simulink model "Position"  (R2021a)
settings: Solver=ode113  StartTime=0.0  StopTime=1  RelTol=1e-6
model workspace (MAT data in the model file):
  Vdc = 30
  f_pwm = 10000
libraries: pid_lib x3, spsControlledVoltageSourceLib x1, spsGroundLib x1, cstblocks x1, spsPermanentMagnetSynchronousMachineLib x1, spsThreePhaseVIMeasurementLib x1, spsUniversalBridgeLib x1, spsTriangleGeneratorLib x1, spspowerguiLib x1
settings Model: SimulationMode=accelerator  Creator=Zzx  LastModifiedBy=Zzx
settings SolverCC: ZeroCrossAlgorithm=Adaptive

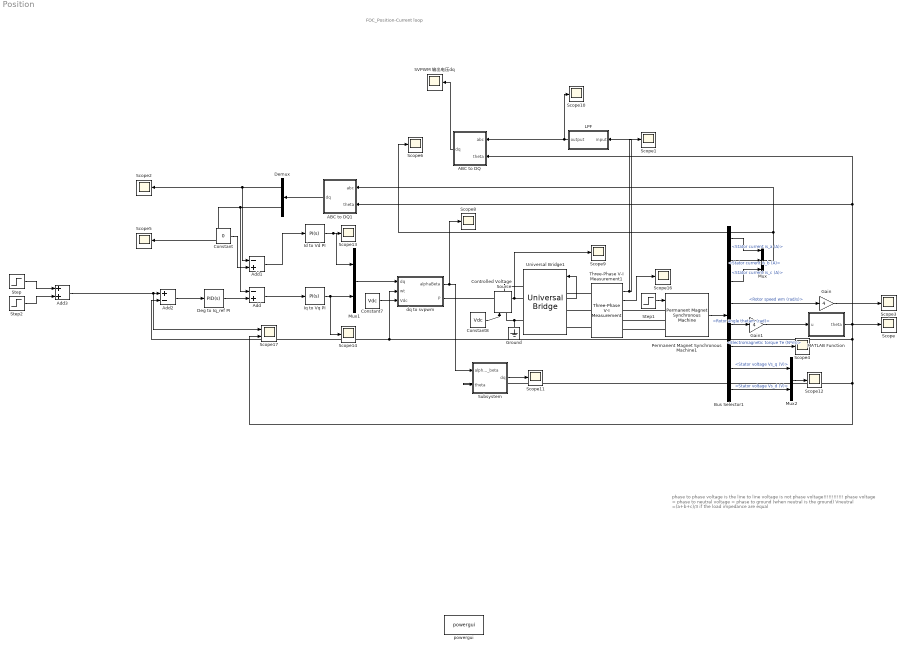
== system Position ==
  note: FOC_Position-Current loop
  note: phase to phase voltage is the line to line voltage
      | is not phase voltage!!!!!!!!!!!!
      | phase voltage = phase to neutral voltage = phase to ground (when neutral is the ground)
      | Vneutral =(a+b+c)/3 if the load impedance are equal
  ABC to DQ : Subsystem
  ABC to DQ1 : Subsystem
  Add : Sum  Inputs=-+
  Add1 : Sum  Inputs=-+
  Add2 : Sum  Inputs=+-
  Add3 : Sum
  Bus Selector1 : BusSelector  OutputSignals=Stator current is_a (A),Stator current is_b (A),Stator current is_c (A),Rotor speed wm (rad/s),Rotor angle thetam (rad),Electromagnetic torque Te (N*m),Stator voltage Vs_q (V),Stator voltage Vs_d (V)
  Constant : Constant  Value=0
  Constant7 : Constant  Value=Vdc
  Constant8 : Constant  Value=Vdc
  Controlled Voltage Source : spsControlledVoltageSourceLib/Controlled Voltage Source  Initialize=on  Source_Type=DC  Amplitude=0  Phase=0  Frequency=0  Measurements=Voltage
  Deg to Iq_ref PI : pid_lib/PID Controller  Controller=PID  Form=Parallel  TimeDomain=Continuous-time  UseExternalTs=off  SampleTime=-1  IntegratorMethod=Forward Euler  FilterMethod=Forward Euler  ControllerParametersSource=internal  P=20  I=0  D=1  UseFilter=on  N=70  TunerSelectOption=Frequency Response Based  InitialConditionSource=internal  InitialConditionForIntegrator=0  InitialConditionForFilter=0  DifferentiatorICPrevScaledInput=0  ExternalReset=none  TrackingMode=off  Kt=1  LimitOutput=off  SatLimitsSource=internal  UpperSaturationLimit=inf  LowerSaturationLimit=-inf  LinearizeAsGain=on  AntiWindupMode=none  Kb=1  POutMin=[]  POutMax=[]  IOutMin=[]  IOutMax=[]  DOutMin=[]  DOutMax=[]  NOutMin=[]  NOutMax=[]  SumOutMin=[]  SumOutMax=[]  SaturationOutMin=[]  SaturationOutMax=[]  PParamMin=[]  PParamMax=[]  IParamMin=[]  IParamMax=[]  DParamMin=[]  DParamMax=[]  NParamMin=[]  NParamMax=[]  KbParamMin=[]  KbParamMax=[]  KtParamMin=[]  KtParamMax=[]  KbOutMin=[]  KbOutMax=[]  KtOutMin=[]  KtOutMax=[]  IntegratorOutMin=[]  IntegratorOutMax=[]  FilterOutMin=[]  FilterOutMax=[]  SumI1OutMin=[]  SumI1OutMax=[]  SumI2OutMin=[]  SumI2OutMax=[]  SumI3OutMin=[]  SumI3OutMax=[]  SumI4OutMin=[]  SumI4OutMax=[]  SumDOutMin=[]  SumDOutMax=[]  DifferentiatorOutMin=[]  DifferentiatorOutMax=[]  FilterDiffOutCoefMin=[]  FilterDiffOutCoefMax=[]  ReciprocalOutMin=[]  ReciprocalOutMax=[]  SumDenOutMin=[]  SumDenOutMax=[]  SumNumOutMin=[]  SumNumOutMax=[]  DivideOutMin=[]  DivideOutMax=[]  UdiffTsProdOutMin=[]  UdiffTsProdOutMax=[]  NTsProdOutMin=[]  NTsProdOutMax=[]  UintegralTsProdOutMin=[]  UintegralTsProdOutMax=[]  UngainTsProdOutMin=[]  UngainTsProdOutMax=[]  IntegratorContinuousStateAttributes=''  IntegratorStateMustResolveToSignalObject=off  IntegratorRTWStateStorageClass=Auto  FilterContinuousStateAttributes=''  FilterStateMustResolveToSignalObject=off  FilterRTWStateStorageClass=Auto  ParallelPVariant=InternalParameters  IdealPVariant=Disabled  IVariant=InternalParameters  DVariant=InternalParameters  IntegratorVariant=Continuous  SatVariant=Disabled  AWVariant=Passthrough  PCopyVariant=Disabled  TRVariant=Disabled  FdbkBlocksVariant=Forward  IdealPFdbkVariant=Disabled  SatFdbkVariant=Disabled  DerivativeFilterVariant=ContFilter  NVariant=InternalParameters  NCopyVariant=Disabled  FilterICVariant=InternalICsFilter  IntegratorICVariant=InternalICs  ExternalResetVariant=Disabled  TRSumVariant=Passthrough  SumFdbkVariant=Disabled  SumVariant=Sum_PID  TsampFilterVariant=InternalTs  TsampNgainVariant=Passthrough  TsampIntegralVariant=Passthrough  ExternalSaturationOutDataTypeStr=Inherit: Same as second input
  Demux : Demux  Outputs=2
  Gain : Gain  Gain=4
  Gain1 : Gain  Gain=4
  Ground : spsGroundLib/Ground  LConnTagsString=a
  Id to Vd PI : pid_lib/PID Controller  Controller=PI  Form=Parallel  TimeDomain=Continuous-time  UseExternalTs=off  SampleTime=-1  IntegratorMethod=Forward Euler  FilterMethod=Forward Euler  ControllerParametersSource=internal  P=10  I=0.1  D=0  UseFilter=on  N=100  TunerSelectOption=Transfer Function Based (PID Tuner App)  InitialConditionSource=internal  InitialConditionForIntegrator=0  InitialConditionForFilter=0  DifferentiatorICPrevScaledInput=0  ExternalReset=none  TrackingMode=off  Kt=1  LimitOutput=off  SatLimitsSource=internal  UpperSaturationLimit=inf  LowerSaturationLimit=-inf  LinearizeAsGain=on  AntiWindupMode=none  Kb=1  POutMin=[]  POutMax=[]  IOutMin=[]  IOutMax=[]  DOutMin=[]  DOutMax=[]  NOutMin=[]  NOutMax=[]  SumOutMin=[]  SumOutMax=[]  SaturationOutMin=[]  SaturationOutMax=[]  PParamMin=[]  PParamMax=[]  IParamMin=[]  IParamMax=[]  DParamMin=[]  DParamMax=[]  NParamMin=[]  NParamMax=[]  KbParamMin=[]  KbParamMax=[]  KtParamMin=[]  KtParamMax=[]  KbOutMin=[]  KbOutMax=[]  KtOutMin=[]  KtOutMax=[]  IntegratorOutMin=[]  IntegratorOutMax=[]  FilterOutMin=[]  FilterOutMax=[]  SumI1OutMin=[]  SumI1OutMax=[]  SumI2OutMin=[]  SumI2OutMax=[]  SumI3OutMin=[]  SumI3OutMax=[]  SumI4OutMin=[]  SumI4OutMax=[]  SumDOutMin=[]  SumDOutMax=[]  DifferentiatorOutMin=[]  DifferentiatorOutMax=[]  FilterDiffOutCoefMin=[]  FilterDiffOutCoefMax=[]  ReciprocalOutMin=[]  ReciprocalOutMax=[]  SumDenOutMin=[]  SumDenOutMax=[]  SumNumOutMin=[]  SumNumOutMax=[]  DivideOutMin=[]  DivideOutMax=[]  UdiffTsProdOutMin=[]  UdiffTsProdOutMax=[]  NTsProdOutMin=[]  NTsProdOutMax=[]  UintegralTsProdOutMin=[]  UintegralTsProdOutMax=[]  UngainTsProdOutMin=[]  UngainTsProdOutMax=[]  IntegratorContinuousStateAttributes=''  IntegratorStateMustResolveToSignalObject=off  IntegratorRTWStateStorageClass=Auto  FilterContinuousStateAttributes=''  FilterStateMustResolveToSignalObject=off  FilterRTWStateStorageClass=Auto  ParallelPVariant=InternalParameters  IdealPVariant=Disabled  IVariant=InternalParameters  DVariant=Disabled  IntegratorVariant=Continuous  SatVariant=Disabled  AWVariant=Passthrough  PCopyVariant=Disabled  TRVariant=Disabled  FdbkBlocksVariant=Forward  IdealPFdbkVariant=Disabled  SatFdbkVariant=Disabled  DerivativeFilterVariant=Disabled  NVariant=Disabled  NCopyVariant=Disabled_SignalSpec  FilterICVariant=Disabled  IntegratorICVariant=InternalICs  ExternalResetVariant=Disabled  TRSumVariant=Passthrough  SumFdbkVariant=Disabled  SumVariant=Sum_PI  TsampFilterVariant=InternalTs  TsampNgainVariant=Passthrough  TsampIntegralVariant=Passthrough  ExternalSaturationOutDataTypeStr=Inherit: Same as second input
  Iq to Vq PI : pid_lib/PID Controller  Controller=PI  Form=Parallel  TimeDomain=Continuous-time  UseExternalTs=off  SampleTime=-1  IntegratorMethod=Forward Euler  FilterMethod=Forward Euler  ControllerParametersSource=internal  P=10  I=0.1  D=0  UseFilter=on  N=100  TunerSelectOption=Frequency Response Based  InitialConditionSource=internal  InitialConditionForIntegrator=0  InitialConditionForFilter=0  DifferentiatorICPrevScaledInput=0  ExternalReset=none  TrackingMode=off  Kt=1  LimitOutput=off  SatLimitsSource=internal  UpperSaturationLimit=inf  LowerSaturationLimit=-inf  LinearizeAsGain=on  AntiWindupMode=none  Kb=1  POutMin=[]  POutMax=[]  IOutMin=[]  IOutMax=[]  DOutMin=[]  DOutMax=[]  NOutMin=[]  NOutMax=[]  SumOutMin=[]  SumOutMax=[]  SaturationOutMin=[]  SaturationOutMax=[]  PParamMin=[]  PParamMax=[]  IParamMin=[]  IParamMax=[]  DParamMin=[]  DParamMax=[]  NParamMin=[]  NParamMax=[]  KbParamMin=[]  KbParamMax=[]  KtParamMin=[]  KtParamMax=[]  KbOutMin=[]  KbOutMax=[]  KtOutMin=[]  KtOutMax=[]  IntegratorOutMin=[]  IntegratorOutMax=[]  FilterOutMin=[]  FilterOutMax=[]  SumI1OutMin=[]  SumI1OutMax=[]  SumI2OutMin=[]  SumI2OutMax=[]  SumI3OutMin=[]  SumI3OutMax=[]  SumI4OutMin=[]  SumI4OutMax=[]  SumDOutMin=[]  SumDOutMax=[]  DifferentiatorOutMin=[]  DifferentiatorOutMax=[]  FilterDiffOutCoefMin=[]  FilterDiffOutCoefMax=[]  ReciprocalOutMin=[]  ReciprocalOutMax=[]  SumDenOutMin=[]  SumDenOutMax=[]  SumNumOutMin=[]  SumNumOutMax=[]  DivideOutMin=[]  DivideOutMax=[]  UdiffTsProdOutMin=[]  UdiffTsProdOutMax=[]  NTsProdOutMin=[]  NTsProdOutMax=[]  UintegralTsProdOutMin=[]  UintegralTsProdOutMax=[]  UngainTsProdOutMin=[]  UngainTsProdOutMax=[]  IntegratorContinuousStateAttributes=''  IntegratorStateMustResolveToSignalObject=off  IntegratorRTWStateStorageClass=Auto  FilterContinuousStateAttributes=''  FilterStateMustResolveToSignalObject=off  FilterRTWStateStorageClass=Auto  ParallelPVariant=InternalParameters  IdealPVariant=Disabled  IVariant=InternalParameters  DVariant=Disabled  IntegratorVariant=Continuous  SatVariant=Disabled  AWVariant=Passthrough  PCopyVariant=Disabled  TRVariant=Disabled  FdbkBlocksVariant=Forward  IdealPFdbkVariant=Disabled  SatFdbkVariant=Disabled  DerivativeFilterVariant=Disabled  NVariant=Disabled  NCopyVariant=Disabled_SignalSpec  FilterICVariant=Disabled  IntegratorICVariant=InternalICs  ExternalResetVariant=Disabled  TRSumVariant=Passthrough  SumFdbkVariant=Disabled  SumVariant=Sum_PI  TsampFilterVariant=InternalTs  TsampNgainVariant=Passthrough  TsampIntegralVariant=Passthrough  ExternalSaturationOutDataTypeStr=Inherit: Same as second input
  LPF : Subsystem
  MATLAB Function : MATLAB Function  TreatAsAtomicUnit=on
  Mux : Mux  Inputs=3
  Mux1 : Mux  Inputs=2
  Mux2 : Mux  Inputs=2
  Permanent Magnet Synchronous Machine1 : spsPermanentMagnetSynchronousMachineLib/Permanent Magnet Synchronous Machine  NbPhases=3  FluxDistribution=Sinusoidal  RotorType=Round  MechanicalLoad=Torque Tm  PresetModel=No  ShowDetailedParameters=on  MeasurementBus=off  Resistance=0.89  Inductance=8.5e-3  dqInductances=[8.5e-3,8.5e-3]  La=0.00062  MachineConstant=Voltage Constant (V_peak L-L / krpm)  Flux=0.0056925  VoltageCst=4.13  TorqueCst=0.034155  Flat=120  Mechanical=[ 0.8e-3, 0 4]  PolePairs=4  InitialConditions=[0,0, 0,0]  InitialConditions5ph=[0 0 0 0 0 0]  RefAngle=Aligned with phase A axis (original Park)  IterativeDiscreteModel=Trapezoidal non iterative  TsBlock=-1  TsPowergui=0
  SVPWM 输出电压dq : Scope
  Scope{,1..6,8..14,16} (15 alike) : Scope
  Scope17 : Scope  NumInputPorts=2
  Step : Step  Time=0.25  Before=1  After=5  SampleTime=0
  Step1 : Step  Time=0.5  After=0  SampleTime=0
  Step2 : Step  Time=0.75  After=-2  SampleTime=0
  Subsystem : Subsystem
  Three-Phase V-I Measurement1 : spsThreePhaseVIMeasurementLib/Three-Phase V-I Measurement  VoltageMeasurement=phase-to-ground  SetLabelV=off  LabelV=Vabc  Vpu=off  VpuLL=off  CurrentMeasurement=yes  SetLabelI=off  LabelI=Iabc  Ipu=off  Pbase=100e6  Vbase=500e3  OutputType=Complex  PhasorSimulation=off  PSBequivalent=0
  Universal Bridge1 : spsUniversalBridgeLib/Universal Bridge  Arms=3  SnubberResistance=1e5  SnubberCapacitance=inf  Device=IGBT / Diodes  Ron=1e-3  Lon=0  ForwardVoltages="[  0  0  ]"  ForwardVoltage=0  GTOparameters=[ 10e-6 , 20e-6 ]  IGBTparameters=[ 1e-6 , 2e-6 ]  Measurements=None  Measurements_2=None  converterType=Rectifier
  dq to svpwm : Subsystem
  powergui : spspowerguiLib/powergui  Priority=1  SimulationMode=Continuous  SampleTime=50e-6  frequency=60  Iterations=50  frequencyindice=0  Pbase=100e6  ErrMax=1e-4  UnitsV=kV  UnitsW=MW  buscounter=0  FunctionMessages=off  echomessages=off  EnableUseOfTLC=off  CurrentSourceSwitches=off  DisableSnubberDevices=off  DisableRonSwitches=off  DisableVfSwitches=off  DisplayEquations=off  AutomaticDiscreteSolvers=off  SolverType=Tustin/Backward Euler (TBE)  Interpol=off  ExternalGateDelay=off  methode=off  Ts=100  x0status=blocks  SPID=on  SwTol=0  HookPort=off  NonlinearTolerance=1e-4  nMaxIteration=100  ContinueOnMaxIteration=off  RestoreLinks=warning  ResistiveCurrentMeasurement=off  Frange=[0:2:500]  Ylog=off  Xlog=on  ShowGrid=off  save=off  variable=ZData  structure=0  ZoomFFT=off  StartTime=0.0  cycles=1  DisplayStyle=1  fundamental=60  FreqAxis=off  MaxFrequency=1000  frequencyindicesteady=1  RmsSteady=1  display=off
  wires:
  Three-Phase V-I Measurement1/1 -> LPF/1(input), Scope1/1
  Permanent Magnet Synchronous Machine1/1 -> Bus Selector1/1
  Bus Selector1/1 -> Mux/1  "<Stator current is_a (A)>"
  Bus Selector1/2 -> Mux/2  "<Stator current is_b (A)>"
  Bus Selector1/3 -> Mux/3  "<Stator current is_c (A)>"
  Mux/1 -> Scope6/1, ABC to DQ1/1(abc)
  Bus Selector1/5 -> Gain1/1  "<Rotor angle thetam (rad)>"
  ABC to DQ1/1(dq) -> Demux/1
  Constant/1 -> Add1/2
  Demux/1 -> Scope2/1, Add1/1
  Demux/2 -> Scope5/1, Add/1
  Bus Selector1/4 -> Gain/1  "<Rotor speed wm (rad/s)>"
  Bus Selector1/6 -> Scope4/1  "<Electromagnetic torque Te (N*m)>"
  Add1/1 -> Id to Vd PI/1
  dq to svpwm/2(P) -> Universal Bridge1/1, Scope9/1
  Mux1/1 -> dq to svpwm/1(dq)
  dq to svpwm/1(alphaBeta) -> Subsystem/1(alpha_beta), Scope8/1
  Bus Selector1/7 -> Mux2/1  "<Stator voltage Vs_q (V)>"
  Bus Selector1/8 -> Mux2/2  "<Stator voltage Vs_d (V)>"
  Mux2/1 -> Scope12/1
  Step1/1 -> Permanent Magnet Synchronous Machine1/1
  Constant7/1 -> dq to svpwm/3(Vdc)
  Three-Phase V-I Measurement1/2 -> Scope16/1
  Constant8/1 -> Controlled Voltage Source/1
  ABC to DQ/1(dq) -> SVPWM 输出电压dq/1
  Id to Vd PI/1 -> Mux1/1, Scope13/1
  Subsystem/1(dq) -> Scope11/1
  LPF/1(output) -> Scope10/1, ABC to DQ/1(abc)
  MATLAB Function/1(theta) -> Scope17/2, Subsystem/2(theta), Add2/2, dq to svpwm/2(wt), ABC to DQ1/2(theta), ABC to DQ/2(theta), Scope/1
  Add3/1 -> Scope17/1, Add2/1
  Step2/1 -> Add3/2
  Step/1 -> Add3/1
  Iq to Vq PI/1 -> Scope14/1, Mux1/2
  Add/1 -> Iq to Vq PI/1
  Gain/1 -> Scope3/1
  Gain1/1 -> MATLAB Function/1(u)
  Deg to Iq_ref PI/1 -> Add/2
  Add2/1 -> Deg to Iq_ref PI/1
  connections:
  Controlled Voltage Source/RConn1 -- Universal Bridge1/RConn1
  Three-Phase V-I Measurement1/LConn1 -- Universal Bridge1/LConn1
  Universal Bridge1/RConn2 -- Controlled Voltage Source/LConn1 -- Ground/LConn1
  Three-Phase V-I Measurement1/LConn3 -- Universal Bridge1/LConn3
  Three-Phase V-I Measurement1/LConn2 -- Universal Bridge1/LConn2
  Permanent Magnet Synchronous Machine1/LConn1 -- Three-Phase V-I Measurement1/RConn1
  Permanent Magnet Synchronous Machine1/LConn2 -- Three-Phase V-I Measurement1/RConn2
  Permanent Magnet Synchronous Machine1/LConn3 -- Three-Phase V-I Measurement1/RConn3

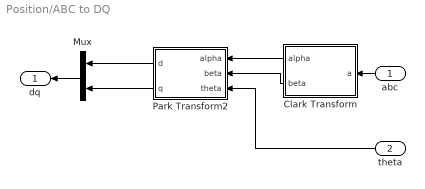
== system Position/ABC to DQ ==
  abc : Inport
  theta : Inport  Port=2
  Clark Transform : MATLAB Function  TreatAsAtomicUnit=on
  Mux : Mux  Inputs=2
  Park Transform2 : MATLAB Function  TreatAsAtomicUnit=on
  dq : Outport
  wires:
  Clark Transform/1(alpha) -> Park Transform2/1(alpha)
  Clark Transform/2(beta) -> Park Transform2/2(beta)
  abc/1 -> Clark Transform/1(a)
  theta/1 -> Park Transform2/3(theta)
  Park Transform2/1(d) -> Mux/1
  Park Transform2/2(q) -> Mux/2
  Mux/1 -> dq/1

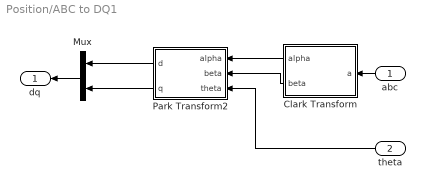
== system Position/ABC to DQ1 ==
  abc : Inport
  theta : Inport  Port=2
  Clark Transform : MATLAB Function  TreatAsAtomicUnit=on
  Mux : Mux  Inputs=2
  Park Transform2 : MATLAB Function  TreatAsAtomicUnit=on
  dq : Outport
  wires:
  Clark Transform/1(alpha) -> Park Transform2/1(alpha)
  Clark Transform/2(beta) -> Park Transform2/2(beta)
  abc/1 -> Clark Transform/1(a)
  theta/1 -> Park Transform2/3(theta)
  Park Transform2/1(d) -> Mux/1
  Park Transform2/2(q) -> Mux/2
  Mux/1 -> dq/1

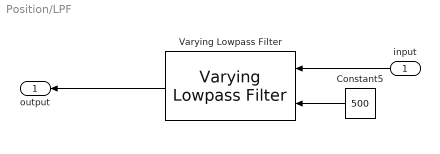
== system Position/LPF ==
  input : Inport
  Constant5 : Constant  Value=500
  Varying Lowpass Filter : cstblocks/Linear Parameter Varying/Varying Lowpass Filter  N=1
  output : Outport
  wires:
  Constant5/1 -> Varying Lowpass Filter/2
  input/1 -> Varying Lowpass Filter/1
  Varying Lowpass Filter/1 -> output/1

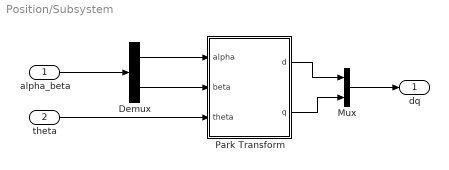
== system Position/Subsystem ==
  alpha_beta : Inport
  theta : Inport  Port=2
  Demux : Demux  Outputs=2
  Mux : Mux  Inputs=2
  Park Transform : MATLAB Function  TreatAsAtomicUnit=on
  dq : Outport
  wires:
  Demux/2 -> Park Transform/2(beta)
  theta/1 -> Park Transform/3(theta)
  Park Transform/1(d) -> Mux/1
  Park Transform/2(q) -> Mux/2
  Mux/1 -> dq/1
  Demux/1 -> Park Transform/1(alpha)
  alpha_beta/1 -> Demux/1

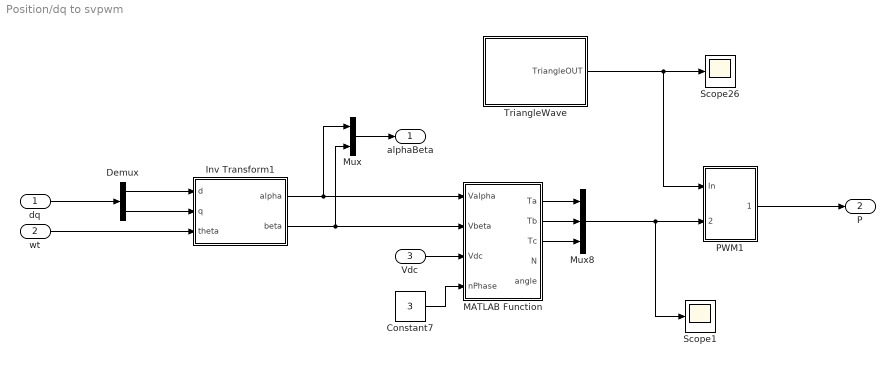
== system Position/dq to svpwm ==
  dq : Inport
  wt : Inport  Port=2
  Vdc : Inport  Port=3
  Constant7 : Constant  Value=3
  Demux : Demux  Outputs=2
  Inv Transform1 : MATLAB Function  TreatAsAtomicUnit=on
  MATLAB Function : MATLAB Function  TreatAsAtomicUnit=on
  Mux : Mux  Inputs=2
  Mux8 : Mux  Inputs=3
  PWM1 : Subsystem
  Scope1 : Scope
  Scope26 : Scope
  TriangleWave : Subsystem
  alphaBeta : Outport
  P : Outport  Port=2
  wires:
  Inv Transform1/2(beta) -> Mux/2, MATLAB Function/2(Vbeta)
  wt/1 -> Inv Transform1/3(theta)
  dq/1 -> Demux/1
  Inv Transform1/1(alpha) -> Mux/1, MATLAB Function/1(Valpha)
  MATLAB Function/1(Ta) -> Mux8/1
  MATLAB Function/3(Tc) -> Mux8/3
  MATLAB Function/2(Tb) -> Mux8/2
  Vdc/1 -> MATLAB Function/3(Vdc)
  Constant7/1 -> MATLAB Function/4(nPhase)
  PWM1/1(PWM) -> P/1
  Mux8/1 -> Scope1/1, PWM1/2(Tcm123)
  Demux/1 -> Inv Transform1/1(d)
  Demux/2 -> Inv Transform1/2(q)
  Mux/1 -> alphaBeta/1
  TriangleWave/1(TriangleOUT) -> Scope26/1, PWM1/1(In)

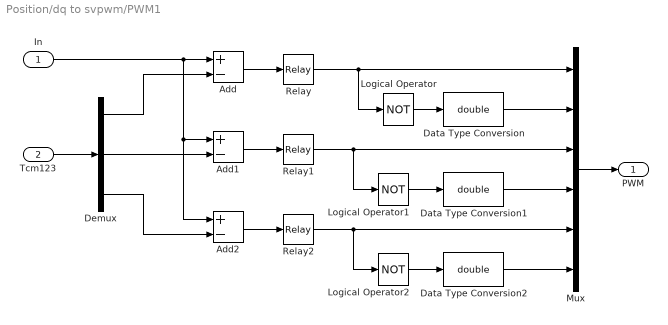
== system Position/dq to svpwm/PWM1 ==
  In : Inport
  Tcm123 : Inport  Port=2
  Add : Sum  Inputs=+-
  Add1 : Sum  Inputs=+-
  Add2 : Sum  Inputs=+-
  Data Type Conversion : DataTypeConversion  OutDataTypeStr=double
  Data Type Conversion1 : DataTypeConversion  OutDataTypeStr=double
  Data Type Conversion2 : DataTypeConversion  OutDataTypeStr=double
  Demux : Demux  Outputs=3
  Logical Operator : Logic  Operator=NOT  AllPortsSameDT=off  OutDataTypeStr=boolean
  Logical Operator1 : Logic  Operator=NOT  AllPortsSameDT=off  OutDataTypeStr=boolean
  Logical Operator2 : Logic  Operator=NOT  AllPortsSameDT=off  OutDataTypeStr=boolean
  Mux : Mux  Inputs=6
  Relay : Relay
  Relay1 : Relay
  Relay2 : Relay
  PWM : Outport
  wires:
  Demux/3 -> Add2/2
  Demux/2 -> Add1/2
  Demux/1 -> Add/2
  Relay2/1 -> Mux/5, Logical Operator2/1
  Relay1/1 -> Mux/3, Logical Operator1/1
  Relay/1 -> Logical Operator/1, Mux/1
  Mux/1 -> PWM/1
  Data Type Conversion/1 -> Mux/2
  Data Type Conversion1/1 -> Mux/4
  Data Type Conversion2/1 -> Mux/6
  Logical Operator2/1 -> Data Type Conversion2/1
  Logical Operator1/1 -> Data Type Conversion1/1
  Logical Operator/1 -> Data Type Conversion/1
  Add1/1 -> Relay1/1
  Add2/1 -> Relay2/1
  Add/1 -> Relay/1
  In/1 -> Add/1, Add2/1, Add1/1
  Tcm123/1 -> Demux/1

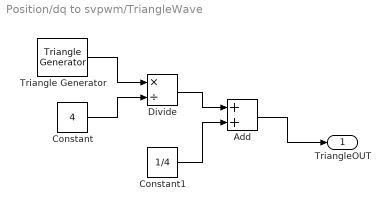
== system Position/dq to svpwm/TriangleWave ==
  Add : Sum
  Constant : Constant  Value=4
  Constant1 : Constant  Value=1/4
  Divide : Product  Inputs=*/
  Triangle Generator : spsTriangleGeneratorLib/Triangle Generator  Freq=f_pwm  Phase=90  Ts=0
  TriangleOUT : Outport
  wires:
  Add/1 -> TriangleOUT/1
  Constant/1 -> Divide/2
  Constant1/1 -> Add/2
  Divide/1 -> Add/1
  Triangle Generator/1 -> Divide/1

== matlab function Position/ABC to DQ/Clark Transform ==
  data: a input; alpha output; beta output
function [alpha,beta] = fcn(a)

alpha = a(1)-0.5*a(2)-0.5*a(3);
beta = 0.5*sqrt(3)*a(2)-0.5*sqrt(3)*a(3);

== matlab function Position/dq to svpwm/MATLAB Function ==
  data: Valpha input; Ta output; Vbeta input; Vdc input; nPhase input; Tb output; Tc output; N output; angle output
function [Ta, Tb, Tc, N,angle ] = FindT(Valpha, Vbeta, Vdc, nPhase)
% from Valpha Vbeta calculates the 
% T0 - the idle time
% T1 - the time at Vi
% T2 - the time at V(i+1) = Vj

nPhase = floor(nPhase);
if nPhase <3
    nPhase = 3;
end

Valpha = Valpha / Vdc;
Vbeta = Vbeta/Vdc;

angle = atan(Vbeta/Valpha);
if Valpha<0
    angle = angle + pi;
end
if angle <0
    angle = angle + 2*pi;
end

i = floor(angle/pi*nPhase);
Vi = exp(1j*pi*i/nPhase);
Vj = exp(1j*pi*(i+1)/nPhase);

Vm = (Vi+Vj)/2;
Vmabs = abs(Vm);
Vout = Valpha + 1j*Vbeta;
%Vabs = abs(Vout);

Vout_para = real(Vout * conj(Vm))/Vmabs;
if Vout_para > Vmabs
    Vout = Vout /Vout_para *Vmabs;
    Vout_para  = Vmabs;
end

T0 = 1- Vout_para / Vmabs;
Vom = Vout / Vout_para *Vmabs - Vm;
T2 = (real(Vom/(Vj-Vi))+0.5) * (1-T0);
T1 = 1-T0-T2;
N = mod(i,2*nPhase);


Tall = [T0/4 T1/2+T0/4 T2/2+T0/4 T1/2+T2/2+T0/4];

switch (N)
case 0
    Ta = Tall(1);
    Tb = Tall(2);
    Tc = Tall(4);
case 1
    Ta = Tall(3);
    Tb = Tall(1);
    Tc = Tall(4);
case 2
    Ta = Tall(4);
    Tb = Tall(1);
    Tc = Tall(2);
case 3
    Ta = Tall(4);
    Tb = Tall(3);
    Tc = Tall(1);
case 4
    Ta = Tall(2);
    Tb = Tall(4);
    Tc = Tall(1);
case 5
    Ta = Tall(1);
    Tb = Tall(4);
    Tc = Tall(3);
otherwise
    Ta = 0;
    Tb = 0;
    Tc = 0;
            
end

end

== matlab function Position/MATLAB Function ==
  data: u input; theta output
function theta = fcn(u)

theta = mod(u,2*pi);

== matlab function Position/dq to svpwm/Inv Transform1 ==
  data: d input; q input; alpha output; theta input; beta output
function [alpha,beta] = fcn(d,q,theta)

alpha = d*cos(theta)-q*sin(theta);
beta = d*sin(theta)+q*cos(theta);

== matlab function Position/ABC to DQ/Park Transform2 ==
  data: alpha input; d output; beta input; theta input; q output
function [d,q] = fcn(alpha,beta,theta)

d = alpha*cos(theta)+beta*sin(theta);
q = -alpha*sin(theta)+beta*cos(theta);

== matlab function Position/ABC to DQ1/Clark Transform ==
  data: a input; alpha output; beta output
function [alpha,beta] = fcn(a)

alpha = a(1)-0.5*a(2)-0.5*a(3);
beta = 0.5*sqrt(3)*a(2)-0.5*sqrt(3)*a(3);

== matlab function Position/ABC to DQ1/Park Transform2 ==
  data: alpha input; d output; beta input; theta input; q output
function [d,q] = fcn(alpha,beta,theta)

d = alpha*cos(theta)+beta*sin(theta);
q = -alpha*sin(theta)+beta*cos(theta);

== matlab function Position/Subsystem/Park Transform ==
  data: alpha input; d output; beta input; theta input; q output
function [d,q] = fcn(alpha,beta,theta)

d = alpha*cos(theta)+beta*sin(theta);
q = -alpha*sin(theta)+beta*cos(theta);
